simulink model "PR_Planar_Testbench_2018"  (R2024a)
settings: Solver=FixedStepDiscrete  StartTime=0.0  StopTime=inf  FixedStep=param.t_sample  RelTol=1e-3
undefined symbols (not defined in the file): max_qa, min_qa, param, slave3
libraries: Cust_Library_planarPKM x54, simulink_extras x27, dspswit3 x24, simulink x22, etherlab_lib x12
(part 6 of 6)

== matlab function PR_Planar_Testbench_2018/Logic/Gradient calculation ==
  data: xEE input; grad output; d_grad output; param parameter
function [grad, d_grad] = grad_3RRR(xEE, param)
    % Funktion für die Bestimmung der korrigierten Plattformsollorientierung zur Strukturöffnung 
    % Eingabe:
    % xEE in m und rad: Ist-Plattformkoordinaten (3x1)
    %
    % Ausgabe:
    % grad: Gradient dqp/dphi(3x1)
    % d_grad: Zeitliche Ableitung des Gradienten dqp/dphi(3x1)
    
    % Aran Mohammad, aran.mohammad@imes.uni-hannover.de, 2022-12
    % (C) Institut für Mechatronische Systeme, Universität Hannover
  beta_j=param.beta_j;
  psi_j=param.psi_j;
  r_fixPlat_j=param.r_fixPlat_j;
  r_mobPlat_j = param.r_mobPlat_j;
  l_all_id = param.l_all_id;

  dq_p_j_dphi_e = [0;0;0];
  jac_q_p = [0;0;0];
  if (xEE(1)>=1 || xEE(2)>=1)
      x_E = 0;
      y_E = 0;
      phi_E = 0;
  else
      x_E = xEE(1);
      y_E = xEE(2);
      phi_E = xEE(3);
  end
  dq_p_j_dphi_e(1) = -(-0.2e1 * (x_E + cos(beta_j(1) + phi_E) * r_mobPlat_j(1) - sin(psi_j(1)) * r_fixPlat_j(1)) * sin(beta_j(1) + phi_E) * r_mobPlat_j(1) + 0.2e1 * (y_E + sin(beta_j(1) + phi_E) * r_mobPlat_j(1) + cos(psi_j(1)) * r_fixPlat_j(1)) * cos(beta_j(1) + phi_E) * r_mobPlat_j(1)) / l_all_id(1) / l_all_id(2) * (-(-l_all_id(1) ^ 2 - l_all_id(2) ^ 2 + (x_E + cos(beta_j(1) + phi_E) * r_mobPlat_j(1) - sin(psi_j(1)) * r_fixPlat_j(1)) ^ 2 + (y_E + sin(beta_j(1) + phi_E) * r_mobPlat_j(1) + cos(psi_j(1)) * r_fixPlat_j(1)) ^ 2) ^ 2 / l_all_id(1) ^ 2 / l_all_id(2) ^ 2 + 0.4e1) ^ (-0.1e1 / 0.2e1);
  dq_p_j_dphi_e(2) = -(-0.2e1 * (x_E + cos(beta_j(2) + phi_E) * r_mobPlat_j(2) - sin(psi_j(2)) * r_fixPlat_j(2)) * sin(beta_j(2) + phi_E) * r_mobPlat_j(2) + 0.2e1 * (y_E + sin(beta_j(2) + phi_E) * r_mobPlat_j(2) + cos(psi_j(2)) * r_fixPlat_j(2)) * cos(beta_j(2) + phi_E) * r_mobPlat_j(2)) / l_all_id(3) / l_all_id(4) * (-(-l_all_id(3) ^ 2 - l_all_id(4) ^ 2 + (x_E + cos(beta_j(2) + phi_E) * r_mobPlat_j(2) - sin(psi_j(2)) * r_fixPlat_j(2)) ^ 2 + (y_E + sin(beta_j(2) + phi_E) * r_mobPlat_j(2) + cos(psi_j(2)) * r_fixPlat_j(2)) ^ 2) ^ 2 / l_all_id(3) ^ 2 / l_all_id(4) ^ 2 + 0.4e1) ^ (-0.1e1 / 0.2e1);
  dq_p_j_dphi_e(3) = -(-0.2e1 * (x_E + cos(beta_j(3) + phi_E) * r_mobPlat_j(3) - sin(psi_j(3)) * r_fixPlat_j(3)) * sin(beta_j(3) + phi_E) * r_mobPlat_j(3) + 0.2e1 * (y_E + sin(beta_j(3) + phi_E) * r_mobPlat_j(3) + cos(psi_j(3)) * r_fixPlat_j(3)) * cos(beta_j(3) + phi_E) * r_mobPlat_j(3)) / l_all_id(5) / l_all_id(6) * (-(-l_all_id(5) ^ 2 - l_all_id(6) ^ 2 + (x_E + cos(beta_j(3) + phi_E) * r_mobPlat_j(3) - sin(psi_j(3)) * r_fixPlat_j(3)) ^ 2 + (y_E + sin(beta_j(3) + phi_E) * r_mobPlat_j(3) + cos(psi_j(3)) * r_fixPlat_j(3)) ^ 2) ^ 2 / l_all_id(5) ^ 2 / l_all_id(6) ^ 2 + 0.4e1) ^ (-0.1e1 / 0.2e1);
  grad = dq_p_j_dphi_e;

  jac_q_p(1) = -(0.2e1 * sin(beta_j(1) + phi_E) ^ 2 * r_mobPlat_j(1) ^ 2 - 0.2e1 * (x_E + cos(beta_j(1) + phi_E) * r_mobPlat_j(1) - sin(psi_j(1)) * r_fixPlat_j(1)) * cos(beta_j(1) + phi_E) * r_mobPlat_j(1) + 0.2e1 * cos(beta_j(1) + phi_E) ^ 2 * r_mobPlat_j(1) ^ 2 - 0.2e1 * (y_E + sin(beta_j(1) + phi_E) * r_mobPlat_j(1) + cos(psi_j(1)) * r_fixPlat_j(1)) * sin(beta_j(1) + phi_E) * r_mobPlat_j(1)) / l_all_id(1) / l_all_id(2) * (-(-l_all_id(1) ^ 2 - l_all_id(2) ^ 2 + (x_E + cos(beta_j(1) + phi_E) * r_mobPlat_j(1) - sin(psi_j(1)) * r_fixPlat_j(1)) ^ 2 + (y_E + sin(beta_j(1) + phi_E) * r_mobPlat_j(1) + cos(psi_j(1)) * r_fixPlat_j(1)) ^ 2) ^ 2 / l_all_id(1) ^ 2 / l_all_id(2) ^ 2 + 0.4e1) ^ (-0.1e1 / 0.2e1) - (-0.2e1 * (x_E + cos(beta_j(1) + phi_E) * r_mobPlat_j(1) - sin(psi_j(1)) * r_fixPlat_j(1)) * sin(beta_j(1) + phi_E) * r_mobPlat_j(1) + 0.2e1 * (y_E + sin(beta_j(1) + phi_E) * r_mobPlat_j(1) + cos(psi_j(1)) * r_fixPlat_j(1)) * cos(beta_j(1) + phi_E) * r_mobPlat_j(1)) ^ 2 / l_all_id(1) ^ 3 / l_all_id(2) ^ 3 * (-(-l_all_id(1) ^ 2 - l_all_id(2) ^ 2 + (x_E + cos(beta_j(1) + phi_E) * r_mobPlat_j(1) - sin(psi_j(1)) * r_fixPlat_j(1)) ^ 2 + (y_E + sin(beta_j(1) + phi_E) * r_mobPlat_j(1) + cos(psi_j(1)) * r_fixPlat_j(1)) ^ 2) ^ 2 / l_all_id(1) ^ 2 / l_all_id(2) ^ 2 + 0.4e1) ^ (-0.3e1 / 0.2e1) * (-l_all_id(1) ^ 2 - l_all_id(2) ^ 2 + (x_E + cos(beta_j(1) + phi_E) * r_mobPlat_j(1) - sin(psi_j(1)) * r_fixPlat_j(1)) ^ 2 + (y_E + sin(beta_j(1) + phi_E) * r_mobPlat_j(1) + cos(psi_j(1)) * r_fixPlat_j(1)) ^ 2);
  jac_q_p(2) = -(0.2e1 * sin(beta_j(2) + phi_E) ^ 2 * r_mobPlat_j(2) ^ 2 - 0.2e1 * (x_E + cos(beta_j(2) + phi_E) * r_mobPlat_j(2) - sin(psi_j(2)) * r_fixPlat_j(2)) * cos(beta_j(2) + phi_E) * r_mobPlat_j(2) + 0.2e1 * cos(beta_j(2) + phi_E) ^ 2 * r_mobPlat_j(2) ^ 2 - 0.2e1 * (y_E + sin(beta_j(2) + phi_E) * r_mobPlat_j(2) + cos(psi_j(2)) * r_fixPlat_j(2)) * sin(beta_j(2) + phi_E) * r_mobPlat_j(2)) / l_all_id(3) / l_all_id(4) * (-(-l_all_id(3) ^ 2 - l_all_id(4) ^ 2 + (x_E + cos(beta_j(2) + phi_E) * r_mobPlat_j(2) - sin(psi_j(2)) * r_fixPlat_j(2)) ^ 2 + (y_E + sin(beta_j(2) + phi_E) * r_mobPlat_j(2) + cos(psi_j(2)) * r_fixPlat_j(2)) ^ 2) ^ 2 / l_all_id(3) ^ 2 / l_all_id(4) ^ 2 + 0.4e1) ^ (-0.1e1 / 0.2e1) - (-0.2e1 * (x_E + cos(beta_j(2) + phi_E) * r_mobPlat_j(2) - sin(psi_j(2)) * r_fixPlat_j(2)) * sin(beta_j(2) + phi_E) * r_mobPlat_j(2) + 0.2e1 * (y_E + sin(beta_j(2) + phi_E) * r_mobPlat_j(2) + cos(psi_j(2)) * r_fixPlat_j(2)) * cos(beta_j(2) + phi_E) * r_mobPlat_j(2)) ^ 2 / l_all_id(3) ^ 3 / l_all_id(4) ^ 3 * (-(-l_all_id(3) ^ 2 - l_all_id(4) ^ 2 + (x_E + cos(beta_j(2) + phi_E) * r_mobPlat_j(2) - sin(psi_j(2)) * r_fixPlat_j(2)) ^ 2 + (y_E + sin(beta_j(2) + phi_E) * r_mobPlat_j(2) + cos(psi_j(2)) * r_fixPlat_j(2)) ^ 2) ^ 2 / l_all_id(3) ^ 2 / l_all_id(4) ^ 2 + 0.4e1) ^ (-0.3e1 / 0.2e1) * (-l_all_id(3) ^ 2 - l_all_id(4) ^ 2 + (x_E + cos(beta_j(2) + phi_E) * r_mobPlat_j(2) - sin(psi_j(2)) * r_fixPlat_j(2)) ^ 2 + (y_E + sin(beta_j(2) + phi_E) * r_mobPlat_j(2) + cos(psi_j(2)) * r_fixPlat_j(2)) ^ 2);
  jac_q_p(3) = -(0.2e1 * sin(beta_j(3) + phi_E) ^ 2 * r_mobPlat_j(3) ^ 2 - 0.2e1 * (x_E + cos(beta_j(3) + phi_E) * r_mobPlat_j(3) - sin(psi_j(3)) * r_fixPlat_j(3)) * cos(beta_j(3) + phi_E) * r_mobPlat_j(3) + 0.2e1 * cos(beta_j(3) + phi_E) ^ 2 * r_mobPlat_j(3) ^ 2 - 0.2e1 * (y_E + sin(beta_j(3) + phi_E) * r_mobPlat_j(3) + cos(psi_j(3)) * r_fixPlat_j(3)) * sin(beta_j(3) + phi_E) * r_mobPlat_j(3)) / l_all_id(5) / l_all_id(6) * (-(-l_all_id(5) ^ 2 - l_all_id(6) ^ 2 + (x_E + cos(beta_j(3) + phi_E) * r_mobPlat_j(3) - sin(psi_j(3)) * r_fixPlat_j(3)) ^ 2 + (y_E + sin(beta_j(3) + phi_E) * r_mobPlat_j(3) + cos(psi_j(3)) * r_fixPlat_j(3)) ^ 2) ^ 2 / l_all_id(5) ^ 2 / l_all_id(6) ^ 2 + 0.4e1) ^ (-0.1e1 / 0.2e1) - (-0.2e1 * (x_E + cos(beta_j(3) + phi_E) * r_mobPlat_j(3) - sin(psi_j(3)) * r_fixPlat_j(3)) * sin(beta_j(3) + phi_E) * r_mobPlat_j(3) + 0.2e1 * (y_E + sin(beta_j(3) + phi_E) * r_mobPlat_j(3) + cos(psi_j(3)) * r_fixPlat_j(3)) * cos(beta_j(3) + phi_E) * r_mobPlat_j(3)) ^ 2 / l_all_id(5) ^ 3 / l_all_id(6) ^ 3 * (-(-l_all_id(5) ^ 2 - l_all_id(6) ^ 2 + (x_E + cos(beta_j(3) + phi_E) * r_mobPlat_j(3) - sin(psi_j(3)) * r_fixPlat_j(3)) ^ 2 + (y_E + sin(beta_j(3) + phi_E) * r_mobPlat_j(3) + cos(psi_j(3)) * r_fixPlat_j(3)) ^ 2) ^ 2 / l_all_id(5) ^ 2 / l_all_id(6) ^ 2 + 0.4e1) ^ (-0.3e1 / 0.2e1) * (-l_all_id(5) ^ 2 - l_all_id(6) ^ 2 + (x_E + cos(beta_j(3) + phi_E) * r_mobPlat_j(3) - sin(psi_j(3)) * r_fixPlat_j(3)) ^ 2 + (y_E + sin(beta_j(3) + phi_E) * r_mobPlat_j(3) + cos(psi_j(3)) * r_fixPlat_j(3)) ^ 2);
  d_grad = jac_q_p;

== matlab function PR_Planar_Testbench_2018/Logic/Clamping reaction ==
  data: grad input; q input; dq input; q_p_min input; xEE_korr output; xEE_soll input; xDEE_soll input; xDDEE_soll input; xDEE_korr output; xDDEE_korr output; xEE_ist input; det_JacA input; det_JacB input; param parameter
function [xEE_korr, xDEE_korr, xDDEE_korr]= klemmgefahr(grad, q, dq, q_p_min, xEE_soll, xDEE_soll, xDDEE_soll, xEE_ist, det_JacA, det_JacB, param)
    % Function for determining the corrected platform target orientation for structure opening 
    % Input:
    % grad: Gradient dqp/dphi(3x1)
    % d_grad: Time derivative of the gradient dqp/dphi(3x1)
    % q in rad: Actual joint coordinates (9x1)
    % dq in rad: Actual joint velocities (9x1)
    % ddq in rad: Actual joint acceleration (9x1)
    % q_p_min in rad: Actual platform speeds (1x1)
    % xEE_soll in m and rad: Target platform coordinates (3x1)
    % xDEE_soll in m/s and rad/s: Target platform speeds (3x1)
    % xDDEE_soll in m/s^2 and rad/s^2: target platform accelerations (3x1)
    %
    % Output:
    % xEE_corr in m and rad: Target platform coordinates with corrected orientation (3x1)
    % xDEE_korr in m/s and rad/s: Target platform speeds with corrected orientation (3x1)
    % xDDEE_korr in m/s^2 and rad/s^2: Target platform accelerations with corrected orientation (3x1)
    % delta_1: Difference between minimum permissible and actual passive angle of the elbow of the first leg chain (1x1)
    % delta_2: Difference between the minimum permissible and actual passive angle of the elbow of the second leg chain (1x1)
    % delta_3: Difference between the minimum permissible and actual passive angle of the elbow of the third leg chain (1x1)

    
    if param.sel_redres == 1
        xEE_korr = xEE_soll;
        xDEE_korr = xDEE_soll;
        xDDEE_korr = xDDEE_soll;
        delta_1 = q(2)-q_p_min;
        delta_2 = q(5)-q_p_min;
        delta_3 = q(8)-q_p_min;
        alpha_rate = 0.01;
         
        [min_dist, ~, ~, ~] = calcShortestDistance(q, param.l_all_id, param.r_fixPlat_j, param.psi_j);

        if param.dmin_SelfColl_m < min_dist && ...
         param.min_det_JacA_hredx < abs(det_JacA) && param.min_det_JacB_hredqa < abs(det_JacB) && ...
         param.max_phie > abs(xEE_ist(3))
          if (delta_1>0)
              xEE_korr(3) = xEE_ist(3) - (delta_1/grad(1))*alpha_rate;
              xDEE_korr(3) = -dq(2)/grad(1)*alpha_rate;
        %       xDDEE_korr(3) = (-ddq(2)-d_grad(1)*xDEE_korr(3))/grad(1);
          elseif (delta_2>0)
              xEE_korr(3) = xEE_ist(3) - (delta_2/grad(2))*alpha_rate;
              xDEE_korr(3) = -dq(5)/grad(2)*alpha_rate;
        %       xDDEE_korr(3) = (-ddq(5)-d_grad(2)*xDEE_korr(3))/grad(2);
          elseif (delta_3>0)
              xEE_korr(3) = xEE_ist(3) - (delta_3/grad(3))*alpha_rate;
              xDEE_korr(3) = -dq(8)/grad(3)*alpha_rate;
        %       xDDEE_korr(3) = (-ddq(8)-d_grad(3)*xDEE_korr(3))/grad(3);
          end
        else
          xEE_korr(3) = xEE_ist(3);
        end
    else
        xEE_korr = zeros(3,1);
        xDEE_korr = zeros(3,1);
        xDDEE_korr = zeros(3,1);
        delta_1 = zeros(1,1);
        delta_2 = zeros(1,1);
        delta_3 = zeros(1,1);
    end

== matlab function PR_Planar_Testbench_2018/Logic/MATLAB Function8 ==
  data: sel_redres input; x output; x_raw input; dx_raw input; ddx_raw input; x_clamping input; dx_clamping input; ddx_clamping input; dx output; ddx output
function [x,dx,ddx] = fcn(sel_redres, x_raw, dx_raw, ddx_raw, ...
                             x_clamping, dx_clamping, ddx_clamping)
    % Function for determining the corrected platform target orientation for structure opening 
    % Input:
    % sel_redres: Gradient dqp/dphi(3x1)
    % x_raw in m and rad: Target platform coordinates (3x1)
    % dx_raw in m and rad: Target platform velocities (3x1)
    % ddx_raw in m and rad: Target platform accelerations (3x1)
    % x_clamping in m and rad: Target platform coordinates for structure opening (3x1)
    % dx_clamping in m and rad: Target platform velocities for structure opening (3x1)
    % ddx_clamping in m and rad: Target platform accelerations for structure opening (3x1)
    % x_sing in m and rad: Target platform coordinates for singularity avoidance (3x1)
    % dx_sing in m/s and rad/s: Target platform velocities for singularity avoidance (3x1)
    % ddx_sing in m/s^2 and rad/s^2: target platform accelerations for singularity avoidance (3x1)
    %
    % Output:
    % x in m and rad: Selected target platform coordinates (3x1)
    % dx in m/s and rad/s: Selected target platform speeds (3x1)
    % ddx in m/s^2 and rad/s^2: Selected target platform accelerations (3x1)
                        
if sel_redres == 1
    x = x_clamping;  
    dx = dx_clamping; 
    ddx = ddx_clamping;    
else    
    x = x_raw;
    dx = dx_raw;
    ddx = ddx_raw;
end

== matlab function PR_Planar_Testbench_2018/Logic/Validation of the EE end target pose/MATLAB Function11 ==
  data: qj_rad input; xEE_ input; qj_soll input; xEE_soll_ input; y output; param parameter
function y = calcJac(qj_rad, xEE_, qj_soll, xEE_soll_, param)
      
      
xEE = [xEE_(1); xEE_(2); 0; 0; 0; xEE_(3)];
xEE_soll = [xEE_soll_(1); xEE_soll_(2); 0; 0; 0; xEE_soll_(3)];

%% individuelle kinematische Parameter
JacA_hredx_ind_3RRRreturn_ist = JacA_hredx_ind_3RRR(qj_rad, xEE, param.l_all_id, param.r_fixPlat_j, param.r_mobPlat_j, param.psi_j, param.beta_j);
JacA_hredx_ind_3RRRreturn_soll = JacA_hredx_ind_3RRR(qj_soll, xEE_soll, param.l_all_id, param.r_fixPlat_j, param.r_mobPlat_j, param.psi_j, param.beta_j);

% Determinanten
prod_det_soll_ist = det(JacA_hredx_ind_3RRRreturn_soll) * det(JacA_hredx_ind_3RRRreturn_ist);

y = prod_det_soll_ist > 0; % Ist das Produkt positiv? Falls ja, dann gibt es keinen Vorzeichenwechsel und damit keine Singularität

== matlab function PR_Planar_Testbench_2018/Logic/Validation of the EE end target pose/komplettes Q über rot ZBen aufstellen ==
  data: qa input; q output; qp input; xEE input; param parameter
function q  = fcn(qa, qp, xEE, param)
phie = xEE(3); 
q13 = phie - (param.psi_j(1) + qa(1) + qp(1)); 
q23 = phie - (param.psi_j(2) + qa(2) + qp(2)); 
q33 = phie - (param.psi_j(3) + qa(3) + qp(3)); 

q = [qa(1); qp(1); q13; ...
    qa(2); qp(2); q23; ...
    qa(3); qp(3); q33];

== matlab function PR_Planar_Testbench_2018/Logic/Safety functions/MATLAB Function3 ==
  data: qj_rad input; y output; param parameter
function y = calcShortestDistance(qj_rad, param)
if param.Exp
    [min_dist, ~, ~, ~] = calcShortestDistance(qj_rad, param.l_all_id, param.r_fixPlat_j, param.psi_j);
    if min_dist > param.dmin_SelfColl_m
        y=false;
    else
        y=true;
    end
else
    y=false;
end

== matlab function PR_Planar_Testbench_2018/Control/MATLAB Function8 ==
  data: kappa output; dkappa output; J_kappa output size=[1,3]; qa_tmp input; q_tmp input; x_tmp input; J_hredxqa_tmp input; J_kappa_prev input; J_dist_prev input; kappa_prev input; mindist_prev input; dJ_kappa output size=[1,3]; min_dist output; dmindist output; J_dist output size=[1,3]; param parameter; dJ_dist output size=[1,3]; det_kappa output; det_mindist output; converged_detLimit_OPspaceLimits_check output
function [kappa, dkappa, J_kappa, dJ_kappa, min_dist, dmindist, J_dist, dJ_dist, det_kappa, det_mindist, converged_detLimit_OPspaceLimits_check] = ...
    fcn(qa_tmp, q_tmp, x_tmp, J_hredxqa_tmp, J_kappa_prev, J_dist_prev, kappa_prev, mindist_prev, param)
    %% Virtuelle Verschiebung im Joint und Task Space
    [q_xtr_virt, q_ytr_virt, q_zrot_virt, x_xtr_virt, x_ytr_virt, x_zrot_virt] = rr_xvirt(x_tmp, param);
    [q_qa1_virt, q_qa2_virt, q_qa3_virt, x_qa1_virt, x_qa2_virt, x_qa3_virt, converged_detLimit_OPspaceLimits_check] = rr_qavirt(qa_tmp, x_tmp, param);
    %% Numerische Berechnung der Jacobi-Matrizen
    [~, kappa, J_kappa, ~, ~] = calcnumJac_kond(J_hredxqa_tmp, q_xtr_virt, q_ytr_virt, q_zrot_virt, x_xtr_virt, x_ytr_virt, x_zrot_virt, ...
                                            q_qa1_virt, q_qa2_virt, q_qa3_virt, x_qa1_virt, x_qa2_virt, x_qa3_virt, param);
    [~,  min_dist, J_dist,  ~,  ~] = calcnumJac_minDist(J_hredxqa_tmp, q_tmp, q_xtr_virt, q_ytr_virt, q_zrot_virt, ...
                                                 q_qa1_virt, q_qa2_virt, q_qa3_virt, param);

    dkappa=(kappa-kappa_prev)*1/param.t_sample;
    dmindist=(min_dist-mindist_prev)*1/param.t_sample;
    dJ_kappa=(reshape(J_kappa,[1,3])-reshape(J_kappa_prev,[1,3]))*1/param.t_sample;
    dJ_dist=(reshape(J_dist,[1,3])-reshape(J_dist_prev,[1,3]))*1/param.t_sample;
    det_kappa = det(J_kappa*J_kappa');
    det_mindist = det(J_dist*J_dist');
end

== matlab function PR_Planar_Testbench_2018/Control/MATLAB Function3 ==
  data: M input; D_d output; K_d input; D input
function D_d=sqrt_damping(M,K_d,D)
%#codegen
K_d1=sqrtm(K_d);
M1 = sqrtm(M);

% if inertia_shaping
D_d_=K_d1*D*M1+M1*D*K_d1;

% assert(max(max(abs(imag(D_d_))))==0, ...
% 'sqrt_damping: Damping Matrix has imaginary parts');
D_d=real(D_d_);

== matlab function PR_Planar_Testbench_2018/Control/MATLAB Function9 ==
  data: alphareact output; rueckzug_aktiv input; rueckzug_aktiv_edge input; tau_in input; tau_out output size=[3,1]; param parameter; tau_prev input
function [alphareact, tau_out] = fcn(rueckzug_aktiv, rueckzug_aktiv_edge, tau_in, param, tau_prev)

persistent alpha_react tau_prereact

if isempty(alpha_react)
    alpha_react = 0;
    tau_prereact = zeros(3,1);
end      

if rueckzug_aktiv_edge
    tau_prereact=tau_prev;
end

if rueckzug_aktiv
%     alphareact = 0.5*tanh(5*alpha_react-2.75)+0.5;
    alphareact=alpha_react;
    alpha_react = alpha_react+param.delta_intermedVal_react;
    if alpha_react>1
        alpha_react=1;
    end
    
    tau_out = alphareact*tau_in + (1-alphareact)*tau_prereact;
else
    alpha_react=0;
    alphareact=0;
    tau_out=tau_in;
end

== matlab function PR_Planar_Testbench_2018/Observer/MATLAB Function5 ==
  data: Fext input; alpha_nf output; nf input; init_reaction input
function alpha_nf = fcn(Fext, nf, init_reaction)
Fx=Fext(1);
Fy=Fext(2);
alpha_nf=0;
    if init_reaction
        alpha_nf = atan2(nf(2), nf(1));
    end
end

== matlab function PR_Planar_Testbench_2018/DirectDynamics_MuJoCo/MATLAB Function5 ==
  data: n input; Fext_link1 output; force_input input size=[4,6]
function Fext_link1  = fcn(n, force_input)
Fext_link1=zeros(3,1);
    if n==1
        Fext_link1 = [force_input(1); force_input(2); force_input(3)];
    end
end

== matlab function PR_Planar_Testbench_2018/Control/MATLAB Function10 ==
  data: u1 input; y output size=[6,1]; u2 input
function y = fcn(u1, u2)
if length(u1)==3 && length(u2)==3
    y = [u1;u2];
elseif length(u1)~=3 && length(u2)==3
    y = [zeros(3,1);u2];
elseif length(u1)==3 && length(u2)~=3
    y = [u1;zeros(3,1)];
else
    y=zeros(6,1);
end

== matlab function PR_Planar_Testbench_2018/Control/MATLAB Function12 ==
  data: kappa_soll output; min_dist_soll output; qa input; q input; x input; param parameter
function [kappa_soll, min_dist_soll] = ...
    fcn(qa, q, x, param)
    %% Virtuelle Verschiebung im Joint und Task Space
    xEE = [x(1); x(2); 0; 0; 0; x(3)];
    JacA_hredx_ind_3RRRreturn = JacA_hredx_ind_3RRR(q, xEE, param.l_all_id, param.r_fixPlat_j, param.r_mobPlat_j, param.psi_j, param.beta_j);
    JacB_hredqa_ind_3RRRreturn = JacB_hredqa_ind_3RRR(q, xEE, param.l_all_id, param.r_fixPlat_j, param.r_mobPlat_j, param.psi_j, param.beta_j);
    Jinv_hredqax_ind_3RRRreturn = -inv(JacB_hredqa_ind_3RRRreturn)*JacA_hredx_ind_3RRRreturn;
    J_hredxqa_tmp = inv(Jinv_hredqax_ind_3RRRreturn);
    [q_xtr_virt, q_ytr_virt, q_zrot_virt, x_xtr_virt, x_ytr_virt, x_zrot_virt] = rr_xvirt(x, param);
    [q_qa1_virt, q_qa2_virt, q_qa3_virt, x_qa1_virt, x_qa2_virt, x_qa3_virt] = rr_qavirt(qa, x, param);
    %% Numerische Berechnung der Jacobi-Matrizen
    [~, kappa_soll, ~, ~, ~] = calcnumJac_kond(J_hredxqa_tmp, q_xtr_virt, q_ytr_virt, q_zrot_virt, x_xtr_virt, x_ytr_virt, x_zrot_virt, ...
                                            q_qa1_virt, q_qa2_virt, q_qa3_virt, x_qa1_virt, x_qa2_virt, x_qa3_virt, param);
    [~,  min_dist_soll, ~,  ~,  ~] = calcnumJac_minDist(J_hredxqa_tmp, q, q_xtr_virt, q_ytr_virt, q_zrot_virt, ...
                                                 q_qa1_virt, q_qa2_virt, q_qa3_virt, param);
end

== matlab function PR_Planar_Testbench_2018/Observer/MATLAB Function6 ==
  data: x input; dx input; q input; dq input; J_xpqa output; J_xpqa_KS0 output; n_f_qa output; Jinv_hqx input; J_hredxqa input; predbody input; predLoc_2D input; predForce_2D input; predLoc_3D input; predForce_3D input; param parameter; n_f_xp output; n_f_xp_KS0 output; qa_sel output; tau_ext input; xp_KS0 output; dxp_KS0 output; xp_KSGj output; dxp_KSGj output; R_0Gj output; dRxp output; dR_0Gj output; q_rad_contact input
function [J_xpqa, J_xpqa_KS0, n_f_qa, n_f_xp, n_f_xp_KS0, qa_sel, xp_KS0, dxp_KS0, xp_KSGj, dxp_KSGj, R_0Gj, dRxp, dR_0Gj]...
    = fcn(x, dx, q, dq, Jinv_hqx, J_hredxqa, predbody, predLoc_2D, predForce_2D, predLoc_3D, predForce_3D, param, tau_ext, q_rad_contact)
    Fext_xp = zeros(3,1);
    Jac_xpq_contact1_ = zeros(3,3);
    dRxp = zeros(2,1);
    R_0Gj=zeros(3,3);
    dR_0Gj=zeros(3,3);
    J_xpqa = zeros(3,3);
    J_xpqa_KS0 = zeros(3,3);
    n_f_qa = zeros(3,1);
    n_f_xp = zeros(3,1);
    n_f_xp_KS0=zeros(3,1);
    xp_KS0 = zeros(3,1);
    dxp_KS0= zeros(3,1);
    xp_KSGj= zeros(3,1);
    dxp_KSGj= zeros(3,1);
    qa_sel = 0;
    if predbody == 1 || predbody == 2
        nr_chain = 1;
    elseif predbody == 3 || predbody == 4
        nr_chain = 2;
    elseif predbody == 5 || predbody == 6
        nr_chain = 3;
    else
        return 
    end
    
    qa = q([1 4 7]);
    dqa = dq([1 4 7]);
    qp = q([2 5 8]);
    dqp = dq([2 5 8]);
    
    qa_contact = q_rad_contact([1 4 7]);
    qp_contact = q_rad_contact([2 5 8]);
    if predbody == 1 || predbody == 3 || predbody == 5
%             qseg = qa(nr_chain) + param.psi_j(nr_chain);  
%             qseg = qa_contact(nr_chain) + param.psi_j(nr_chain);  
%             dqseg = dqa(nr_chain);    
%             [~, ~, ~, Jac_xpq_contact1_, ~, ~, ~, ~, dxp_KS0, xp_KS0]... 
%                 = calcJac_colSeg(1, q, dq, x, dx, param.l_all, param.r_BasisPla_MobPla, ...
%                                  param.l_all_id, param.r_fixPlat_j, param.r_mobPlat_j, nr_chain, 0.5, 0);
            J_xpqa = zeros(3,3);
            J_xpqa(1, nr_chain) = 1;
            n_f_qa = zeros(3,1);
            n_f_qa(nr_chain) = 1*sign(tau_ext(nr_chain));
            qa_sel = qa_contact(nr_chain);
            
            
%             Fext_xp = [0; tau_ext(nr_chain)/l;0];
%             r_0Gj_KS0 = [sin(param.psi_j(nr_chain));  -cos(param.psi_j(nr_chain))]*param.r_fixPlat_j(nr_chain); % Inertial zu Basisgelenk 1
    elseif predbody == 2 || predbody == 4 || predbody == 6 
%         qseg = qa(nr_chain) + param.psi_j(nr_chain)+qp(nr_chain);    
        qseg = qa_contact(nr_chain) + param.psi_j(nr_chain)+qp_contact(nr_chain);    
%         dqseg = dqa(nr_chain) + dqp(nr_chain);  
        if param.pf_dim == 2
            [~, ~, ~, Jac_xpq_contact1_, ~, ~, ~, ~, dxp_KS0, xp_KS0]... 
                = calcJac_colSeg(2, q, dq, x, dx, param.l_all, param.r_BasisPla_MobPla, ...
                                 param.l_all_id, param.r_fixPlat_j, param.r_mobPlat_j, nr_chain, predLoc_2D, 0);
            Fext_xp = [0; predForce_2D;0];
        elseif param.pf_dim == 3
            [~, ~, ~, Jac_xpq_contact1_, ~, ~, ~, ~, dxp_KS0, xp_KS0]... 
                = calcJac_colSeg(2, q, dq, x, dx, param.l_all, param.r_BasisPla_MobPla, ...
                                 param.l_all_id, param.r_fixPlat_j, param.r_mobPlat_j, nr_chain, predLoc_3D, 0);
            Fext_xp = [predForce_3D(1); predForce_3D(2);0];
        end
        r_0Gj_KS0 = [sin(param.psi_j(nr_chain));                -cos(param.psi_j(nr_chain))]*param.r_fixPlat_j(nr_chain)+...% Inertial zu Basisgelenk 1
                    [cos(param.psi_j(nr_chain) + qa(nr_chain));  sin(param.psi_j(nr_chain)  + qa(nr_chain))]*param.l_all_id(nr_chain*2-1);% Basisgelenk1 zu Elle 1
        R_0Gj = [cos(qseg) -sin(qseg) 0 ; sin(qseg) cos(qseg) 0 ;0 0 1]; 
%         dR_0Gj = calcTimeDerivRot(qseg, dqseg);
        xp_KSGj = xp_KS0;
%         xp_KSGj(1:2) = R_0Gj(1:2,1:2)'*(xp_KS0(1:2)-r_0Gj_KS0);
        xp_KSGj(1:2) = R_0Gj(1:2,1:2)'*xp_KS0(1:2);
        dxp_KSGj = dxp_KS0;
%         dRxp = dR_0Gj(1:2,1:2)*xp_KS0(1:2);
        dxp_KSGj(1:2) = R_0Gj(1:2,1:2)'*dxp_KS0(1:2)+dRxp*0;    
        Jac_xpq_contact1 = Jac_xpq_contact1_;
        Jac_xpq_contact1(1:2,:) = R_0Gj(1:2,1:2)'*Jac_xpq_contact1(1:2,:);
        J_xpx_contact = Jac_xpq_contact1 * Jinv_hqx;
        J_xpqa = J_xpx_contact*J_hredxqa;
        J_xpqa_KS0 = J_xpqa;
        J_xpqa_KS0(1:2,:) = R_0Gj(1:2,1:2)*J_xpqa(1:2,:);
        Fext_xp_KS0=zeros(3,1);
        Fext_xp_KS0(1:2)=R_0Gj(1:2,1:2)*Fext_xp(1:2,1);

        if norm(Fext_xp(1:3))<1e-3
            n_f_xp =Fext_xp(1:3)/(norm(Fext_xp(1:3))+1e-3); % Richtungsvektor der Geraden (Verschiebung der Kraft entlang der Wirklinie)
        else
            n_f_xp =Fext_xp(1:3)/norm(Fext_xp(1:3)); % Richtungsvektor der Geraden (Verschiebung der Kraft entlang der Wirklinie)
        end

        if norm(Fext_xp_KS0(1:3))<1e-3
            n_f_xp_KS0 =Fext_xp_KS0(1:3)/(norm(Fext_xp_KS0(1:3))+1e-3); % Richtungsvektor der Geraden (Verschiebung der Kraft entlang der Wirklinie)
        else
            n_f_xp_KS0 =Fext_xp_KS0(1:3)/norm(Fext_xp_KS0(1:3)); % Richtungsvektor der Geraden (Verschiebung der Kraft entlang der Wirklinie)
        end
    end    
end

function dRz = calcTimeDerivRot(phi, dphi)
    cphi = cos(phi);
    sphi = sin(phi);
    dRz = [-sphi*dphi -cphi*dphi 0;
            cphi*dphi -sphi*dphi 0;
            0          0         0];
end

== matlab function PR_Planar_Testbench_2018/DirectDynamics_MuJoCo/Planare PKM ==
  data: tau input; q output; qd output; qdd output
function [q, qd, qdd] = call_mujoco(tau)
    % Funktion für den Mujoco-Aufruf und -Ausgabe der kinematischen Größen
    % Eingabe:
    % tau in Nm: Antriebsmomente in Antriebskoordinaten (3x1)
    %
    % Ausgabe:
    % q_ in m und rad: Vektor der Gelenk- und Plattformkoordinaten (12x1)
    % qd_ in m/s und rad/s: Vektor der Gelenk- und Plattformgeschwindigkeiten (12x1)
    % qdd_ in m/s^2 und rad/s^2: Vektor der Gelenk- und Plattformbeschleunigungen (12x1)
    
    % Aran Mohammad, aran.mohammad@imes.uni-hannover.de, 2022-12
    % (C) Institut für Mechatronische Systeme, Universität Hannover
%#codegen
coder.extrinsic('mjx');
coder.extrinsic('evalin');
mjx('set', 'ctrl', tau');

mjx('step', param.t_sample/0.001);

q_ = zeros(12,1); 
qd = zeros(12,1); 
qdd = zeros(12,1);

qoffset =[25.5184; 122.3049; -237.8233; ...
     0; 0; 0; ...
     25.9632; 121.7747; -358.5010; ...
     24.3787; 124.6086; -479.4775]*pi/180;

q_ = mjx('get', 'qpos');
q = q_ + qoffset;
qd = mjx('get', 'qvel');
qdd = mjx('get', 'qacc');

== matlab function PR_Planar_Testbench_2018/Logic/MATLAB Function14 ==
  data: Init_Reaktion input; x_soll_retr_m_rad output; n_f input; x_ist input; d_rueckz_m input; qa_contact_sel_rad input; predbody input; n_f_qa input; x_ist_retr output
function [x_soll_retr_m_rad, x_ist_retr] = fcn(Init_Reaktion, n_f, x_ist, d_rueckz_m, qa_contact_sel_rad, predbody, n_f_qa)
    if Init_Reaktion
        nr_chain=1;
        x_ist_retr=x_ist;
        delta_x=zeros(3,1);
        if predbody == 1 || predbody == 2
            nr_chain = 1;
        elseif predbody == 3 || predbody == 4
            nr_chain = 2;
        elseif predbody == 5 || predbody == 6
            nr_chain = 3;
        end
        if predbody==1 || predbody==3 || predbody==5
             
            delta_x = [n_f_qa(1)*d_rueckz_m/0.5; n_f_qa(2)*d_rueckz_m/0.5; n_f_qa(3)*d_rueckz_m/0.5];
            x_ist_retr=zeros(3,1);
            x_ist_retr(nr_chain) = qa_contact_sel_rad;
            
        elseif  predbody==2 || predbody==4 || predbody==6
            
            delta_x = [n_f(1)*d_rueckz_m; n_f(2)*d_rueckz_m; 0];
            x_ist_retr = x_ist;
            
        end
        x_soll_retr_m_rad = x_ist_retr + delta_x;
    else
        x_ist_retr = x_ist;
        x_soll_retr_m_rad = x_ist; 
    end
end

== matlab function PR_Planar_Testbench_2018/Logic/MATLAB Function15 ==
  data: s_in input; v_in input; a_in input; trigger input; s_out output; v_out output; a_out output
function [s_out,v_out,a_out] = fcn(s_in, v_in, a_in, trigger)
    persistent s v a
    n=length(s_in);
    if length(s_in) ==1 || length(v_in) ==1 || length(a_in) ==1
        s_out = zeros(3,1);
        v_out = zeros(3,1);
        a_out = zeros(3,1);
        return
    end
    if isempty(s)
        s = s_in;
        v = v_in;
        a = a_in;
    end
    if trigger == 1
        s = s_in;
        v = v_in;
        a = a_in;
    end
    s_out = s;
    v_out = v;
    a_out = a;
end

== matlab function PR_Planar_Testbench_2018/Logic/MATLAB Function16 ==
  data: n_f_xp input; n_f_xp_sel output; n_f_xp_KS0 input; xp_KSGj input; xp_KS0 input; xp_sel output; rueck_KS0 input
function [n_f_xp_sel, xp_sel] = fcn(n_f_xp, n_f_xp_KS0, xp_KSGj, xp_KS0, rueck_KS0)
    if rueck_KS0 == 2 
        n_f_xp_sel = n_f_xp;
        xp_sel = xp_KSGj;
    else
        n_f_xp_sel = n_f_xp_KS0;
        xp_sel = xp_KS0;
    end

== matlab function PR_Planar_Testbench_2018/Control/MATLAB Function13 ==
  data: u input; y output size=[12,1]; data input; data1 input; data2 input
function y = fcn(u, data, data1, data2)

y = [u;data;data1;data2];

== matlab function PR_Planar_Testbench_2018/Logic/MATLAB Function23 ==
  data: s_in input; v_in input; a_in input; trigger input; s_out output; v_out output; a_out output
function [s_out,v_out,a_out] = fcn(s_in, v_in, a_in, trigger)
    persistent s v a
    n=length(s_in);
    if length(s_in) ==1 || length(v_in) ==1 || length(a_in) ==1
        s_out = zeros(2,1);
        v_out = zeros(2,1);
        a_out = zeros(2,1);
        return
    end
    if isempty(s)
        s = s_in;
        v = v_in;
        a = a_in;
    end
    if trigger == 1
        s = s_in;
        v = v_in;
        a = a_in;
    end
    s_out = s;
    v_out = v;
    a_out = a;
end

== matlab function PR_Planar_Testbench_2018/Visualization/MATLAB Function2 ==
  data: predLocation_2D input; predLoc output; predContactForce_2D input; predLocation_3D input; predContactForce_3D input; predF output; param parameter
function [predLoc, predF] = fcn(predLocation_2D, predContactForce_2D, predLocation_3D, predContactForce_3D, param)
predLoc = 0;
predF = [0; 0];
if param.pf_dim == 2
   predLoc = predLocation_2D;
   predF = [0; predContactForce_2D];
elseif param.pf_dim == 3
   predLoc = predLocation_3D;
   predF = reshape(predContactForce_3D, [2 1]);    
end

== matlab function PR_Planar_Testbench_2018/Logic/MATLAB Function17 ==
  data: mode input; y output; mode_prev input
function y = fcn(mode, mode_prev)
if (mode == 2 || mode == 4) && mode ~= mode_prev && (mode_prev~=2 && mode_prev~=4) && mode_prev==1
    y = 1;
else
    y=0;
end

== matlab function PR_Planar_Testbench_2018/DirectDynamics_MuJoCo/MATLAB Function1 ==
  data: q_ input; q output; dq_ input; ddq_ input; dq output; ddq output; x output; dx output; ddx output; qcaps output
function [q, dq, ddq, x, dx, ddx, qcaps] = fcn(q_, dq_, ddq_)
    % Funktion für die Sortierung der Mujoco-Größen
    % Eingabe:
    % q_ in m und rad: Vektor der Kapsel-, Gelenk- und Plattformkoordinaten (14x1)
    % qd_ in m/s und rad/s: Vektor der Kapsel-, Gelenk- und Plattformgeschwindigkeiten (14x1)
    % qdd_ in m/s^2 und rad/s^2: Vektor der Kapsel-, Gelenk- und Plattformbeschleunigungen (14x1)
    %
    % Ausgabe:
    % q in rad: Vektor der Plattformkoordinaten (9x1)
    % dq in rad/s: Vektor der Plattformgeschwindigkeiten (9x1)
    % ddq in rad/s^2: Vektor der Plattformbeschleunigungen (9x1)
    % x in m und rad: Vektor der Plattformkoordinaten (3x1)
    % dx in m/s und rad/s: Vektor der Plattformgeschwindigkeiten (3x1)
    % ddx in m/s^2 und rad/s^2: Vektor der Plattformbeschleunigungen (3x1)
    % qcaps in m: Vektor der Kapselkoordinaten (2x1)
    
    % Aran Mohammad, aran.mohammad@imes.uni-hannover.de, 2022-12
    % (C) Institut für Mechatronische Systeme, Universität Hannover

qcaps = q_([1 2]) + [0.4; 0.3];
q = q_([3 4 5 9 10 11 12 13 14]);
x = q_([6 7 8]);

dq = dq_([3 4 5 9 10 11 12 13 14]);
dx = dq_([6 7 8]);

ddq = ddq_([3 4 5 9 10 11 12 13 14]);
ddx = ddq_([6 7 8]);

== matlab function PR_Planar_Testbench_2018/Logic/MATLAB Function18 ==
  data: mode input; y output; mode_prev input
function y = fcn(mode, mode_prev)
if (mode == 3 || mode == 4) && mode ~= mode_prev && (mode_prev~=3 && mode_prev~=4)% && mode_prev==1
    y = 1;
else
    y=0;
end

== matlab function PR_Planar_Testbench_2018/Logic/MATLAB Function19 ==
  data: s_in input; v_in input; a_in input; trigger input; out output
function out  = fcn(s_in, v_in, a_in, trigger)
    persistent s v a
    if isempty(s)
        s = s_in;
        v = v_in;
        a = a_in;
    end
    if trigger == 1
        s = s_in;
        v = v_in;
        a = a_in;
    end
    s_out = s;
    v_out = v;
    a_out = a;
    out = [s_out; v_out; a_out];
end

== matlab function PR_Planar_Testbench_2018/Logic/MATLAB Function20 ==
  data: s_in input; v_in input; a_in input; trigger input; out output
function out  = fcn(s_in, v_in, a_in, trigger)
    persistent s v a
    if isempty(s)
        s = s_in;
        v = v_in;
        a = a_in;
    end
    if trigger == 1
        s = s_in;
        v = v_in;
        a = a_in;
    end
    s_out = s;
    v_out = v;
    a_out = a;
    out = [s_out; v_out; a_out];
end

== matlab function PR_Planar_Testbench_2018/Control/TP1_impl9/MATLAB Function16 ==
  data: u_raw input; u_filt output; u_prev_ input; a input; y_prev_ input; not_defined_nan output
function  [u_filt, not_defined_nan] = TP1_DiffEq(u_raw, u_prev_, a, y_prev_)
y_prev = reshape(y_prev_, [1,3]);
u_prev = reshape(u_prev_, [1,3]);
if isnan(sum(u_raw)) || isinf(sum(u_raw))
    u_filt = zeros(1,3);
    not_defined_nan = 1;
elseif isnan(sum(TP1_DiffEq(u_raw, u_prev, a, y_prev))) || isinf(sum(TP1_DiffEq(u_raw, u_prev, a, y_prev)))
        u_filt = zeros(1,3);
        not_defined_nan = 2;
else
    u_filt = TP1_DiffEq(u_raw, u_prev, a, y_prev);
    not_defined_nan = 0;
end

== matlab function PR_Planar_Testbench_2018/Control/TP1_impl10/MATLAB Function16 ==
  data: u_raw input; u_filt output; u_prev_ input; a input; y_prev_ input; not_defined_nan output
function  [u_filt, not_defined_nan] = TP1_DiffEq(u_raw, u_prev_, a, y_prev_)
y_prev = reshape(y_prev_, [1,3]);
u_prev = reshape(u_prev_, [1,3]);
if isnan(sum(u_raw)) || isinf(sum(u_raw))
    u_filt = zeros(1,3);
    not_defined_nan = 1;
elseif isnan(sum(TP1_DiffEq(u_raw, u_prev, a, y_prev))) || isinf(sum(TP1_DiffEq(u_raw, u_prev, a, y_prev)))
        u_filt = zeros(1,3);
        not_defined_nan = 2;
else
    u_filt = TP1_DiffEq(u_raw, u_prev, a, y_prev);
    not_defined_nan = 0;
end

== matlab function PR_Planar_Testbench_2018/Logic/MATLAB Function21 ==
  data: s_in_ input; v_in_ input; a_in_ input; trigger input; s_out output; v_out output; a_out output; retr_soll output
function [s_out,v_out,a_out, retr_soll] = fcn(s_in_, v_in_, a_in_, trigger)
    
    persistent s v a
%     n=length(s_in);
    s_out = zeros(3,1);
    v_out = zeros(3,1);
    a_out = zeros(3,1);
    retr_soll = zeros(9,1); 
    if length(s_in_) ~=3 || length(v_in_) ~=3 || length(a_in_) ~=3       
        s_in = zeros(3,1);
        v_in = zeros(3,1);
        a_in = zeros(3,1);
        retr_soll = zeros(9,1); 
    else
        s_in = s_in_;
        v_in = v_in_;
        a_in = a_in_;        
    end
    if isempty(s)
        s = zeros(3,1);
        v = zeros(3,1);
        a = zeros(3,1);
    end
    if trigger == 1 && length(s_in) ==3 && length(v_in) ==3 && length(a_in) ==3
        s = s_in;
        v = v_in;
        a = a_in;
    end
    s_out = s;
    v_out = v;
    a_out = a;
    if length(s_in) ==3 && length(v_in) ==3 && length(a_in) ==3
        retr_soll = [s_out; v_out; a_out];
    else
        retr_soll = zeros(9,1);            
    end
end

== matlab function PR_Planar_Testbench_2018/Visualization/MATLAB Function3 ==
  data: u input; y output
function y = fcn(u)

y = norm(u(1:3));

== matlab function PR_Planar_Testbench_2018/Visualization/TP1_impl/MATLAB Function16 ==
  data: u_raw input; u_filt output; u_prev input; a input; y_prev input; not_defined_nan output
function  [u_filt, not_defined_nan] = TP1_DiffEq(u_raw, u_prev, a, y_prev)
if isnan(sum(u_raw))
    u_filt = [0;0;0];
    not_defined_nan = 1;
elseif isnan(sum(TP1_DiffEq(u_raw, u_prev, a, y_prev)))
        u_filt = [0;0;0];
        not_defined_nan = 2;
else
    u_filt = TP1_DiffEq(u_raw, u_prev, a, y_prev);
    not_defined_nan = 0;
end

== matlab function PR_Planar_Testbench_2018/Kinematics/MATLAB Function13 ==
  data: u input; y output; N input
function y = fcn(u, N)
y=N*floor(u/N);

== matlab function PR_Planar_Testbench_2018/Kinematics/MATLAB Function14 ==
  data: qj_rad input; det_JacA_hredx output; det_JacB_hredqa output; xEE_ input; param parameter; cond_J_hredxqa_ind output
function [det_JacA_hredx, det_JacB_hredqa, cond_J_hredxqa_ind] = fcn(qj_rad, xEE_, param)
xEE = [xEE_(1); xEE_(2); 0; 0; 0; xEE_(3)];
JacA_hredx_ind_3RRRreturn = JacA_hredx_ind_3RRR(qj_rad, xEE, param.l_all_id, param.r_fixPlat_j, param.r_mobPlat_j, param.psi_j, param.beta_j);
JacB_hredqa_ind_3RRRreturn = JacB_hredqa_ind_3RRR(qj_rad, xEE, param.l_all_id, param.r_fixPlat_j, param.r_mobPlat_j, param.psi_j, param.beta_j);
% Determinanten
det_JacA_hredx = det(JacA_hredx_ind_3RRRreturn);
det_JacB_hredqa = det(JacB_hredqa_ind_3RRRreturn);


Jinv_hredqax_ind_3RRRreturn = -inv(JacB_hredqa_ind_3RRRreturn)*JacA_hredx_ind_3RRRreturn;
J_hredxqa_ind_3RRRreturn = inv(Jinv_hredqax_ind_3RRRreturn);
cond_J_hredxqa_ind = cond(J_hredxqa_ind_3RRRreturn,2);
